simulink model "self_balancing_slink"  (R2023b)
settings: Solver=ode45  StartTime=0.0  StopTime=10.0  FixedStep=0.01  RelTol=0.001
values from neighbouring files (symbols this model uses):
  dt = 0.01    [bot_main.m]    (also in modelStateTransitionFcn.m)
  g = 9.81    [bot_main.m]    (also in eq_states.m; modelStateTransitionFcn.m)
  I_pend = 0.055    [bot_main.m]    (also in eq_states.m; modelStateTransitionFcn.m)
  Kd = Kg_d(i)    [bot_main.m]
  Ki = Kg_i(i)    [bot_main.m]
  Kp = Kg_p(i)    [bot_main.m]
  l = 0.159    [bot_main.m]    (also in eq_states.m; modelStateTransitionFcn.m)
  m_cart = 0.558    [bot_main.m]    (also in eq_states.m; modelStateTransitionFcn.m)
  m_pend = 1.267    [bot_main.m]    (also in eq_states.m; modelStateTransitionFcn.m)
  mu_drag = 0.00002    (= 2e-05)    [bot_main.m]    (also in eq_states.m = 0.2; modelStateTransitionFcn.m)
  noise_s1_value = np1(i)    [bot_main.m]
  noise_s2_value = np2(i)    [bot_main.m]
  x_init = [0; 0; (11/12)*pi; 0]    [bot_main.m]
libraries: simulink x4, slpidlib x2, sharedTrackingLibrary x2
settings Model: Creator=goate  LastModifiedBy=goate
settings SolverCC: ConsecutiveZCsStepRelTol=2.8421709430404e-13

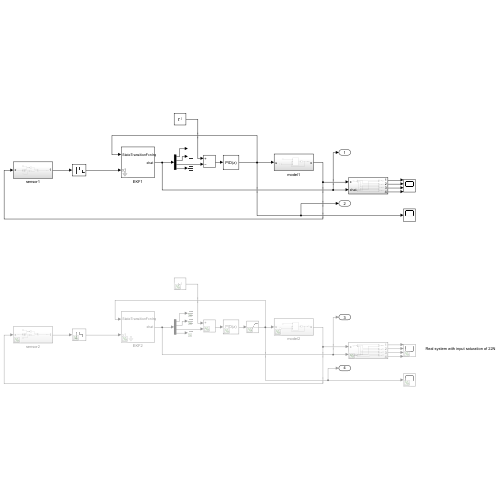
[thumbnail: Simulink's stored preview of the top-level diagram]
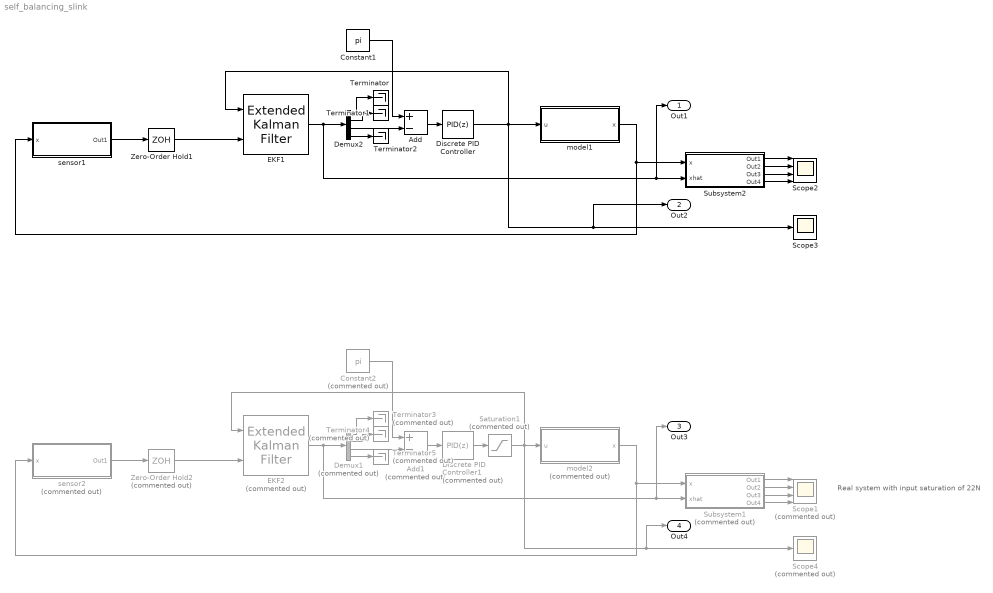
== system self_balancing_slink ==
  note: Real system with input saturation of 22N
  Add : Sum  Inputs=+-
  Add1 : Sum  Commented=on  Inputs=+-
  Constant1 : Constant  Value=pi
  Constant2 : Constant  Commented=on  Value=pi
  Demux1 : Demux  Commented=on
  Demux2 : Demux
  Discrete PID Controller : slpidlib/PID Controller  Controller=PID  Form=Parallel  TimeDomain=Discrete-time  UseExternalTs=off  SampleTime=dt  IntegratorMethod=Forward Euler  FilterMethod=Forward Euler  ControllerParametersSource=internal  P=Kp  I=Ki  UseKiTs=off  D=Kd  N=100  UseFilter=on  TunerSelectOption=Frequency Response Based  InitialConditionSource=internal  InitialConditionForIntegrator=0  InitialConditionForFilter=0  DifferentiatorICPrevScaledInput=0  ExternalReset=none  TrackingMode=off  Kt=1  LimitOutput=off  SatLimitsSource=internal  UpperSaturationLimit=inf  LowerSaturationLimit=-inf  LinearizeAsGain=off  AntiWindupMode=none  Kb=1  LimitIntegrator=off  UpperIntegratorSaturationLimit=inf  LowerIntegratorSaturationLimit=-inf  POutMin=[]  POutMax=[]  IOutMin=[]  IOutMax=[]  DOutMin=[]  DOutMax=[]  NOutMin=[]  NOutMax=[]  SumOutMin=[]  SumOutMax=[]  SaturationOutMin=[]  SaturationOutMax=[]  PParamMin=[]  PParamMax=[]  IParamMin=[]  IParamMax=[]  DParamMin=[]  DParamMax=[]  NParamMin=[]  NParamMax=[]  KbParamMin=[]  KbParamMax=[]  KtParamMin=[]  KtParamMax=[]  KbOutMin=[]  KbOutMax=[]  KtOutMin=[]  KtOutMax=[]  IntegratorOutMin=[]  IntegratorOutMax=[]  FilterOutMin=[]  FilterOutMax=[]  SumI1OutMin=[]  SumI1OutMax=[]  SumI2OutMin=[]  SumI2OutMax=[]  SumI3OutMin=[]  SumI3OutMax=[]  SumI4OutMin=[]  SumI4OutMax=[]  SumDOutMin=[]  SumDOutMax=[]  DifferentiatorOutMin=[]  DifferentiatorOutMax=[]  FilterDiffOutCoefMin=[]  FilterDiffOutCoefMax=[]  ReciprocalOutMin=[]  ReciprocalOutMax=[]  SumDenOutMin=[]  SumDenOutMax=[]  SumNumOutMin=[]  SumNumOutMax=[]  DivideOutMin=[]  DivideOutMax=[]  UdiffTsProdOutMin=[]  UdiffTsProdOutMax=[]  NTsProdOutMin=[]  NTsProdOutMax=[]  UintegralTsProdOutMin=[]  UintegralTsProdOutMax=[]  UngainTsProdOutMin=[]  UngainTsProdOutMax=[]  ClampingZeroOutDataTypeStr=Inherit: Inherit via back propagation  ClampingZeroOutMin=[]  ClampingZeroOutMax=[]  FilterDenConstantOutDataTypeStr=Inherit: Inherit via back propagation  FilterDenConstantOutMin=[]  FilterDenConstantOutMax=[]  PCopyOutDataTypeStr=Inherit: Inherit via back propagation  PCopyOutMin=[]  PCopyOutMax=[]  NCopyOutDataTypeStr=Inherit: Inherit via back propagation  NCopyOutMin=[]  NCopyOutMax=[]  IntegratorContinuousStateAttributes=''  IntegratorStateMustResolveToSignalObject=off  IntegratorRTWStateStorageClass=Auto  FilterContinuousStateAttributes=''  FilterStateMustResolveToSignalObject=off  FilterRTWStateStorageClass=Auto  ParallelPVariant=InternalParameters  IdealPVariant=Disabled  IVariant=InternalParameters  DVariant=InternalParameters  IntegratorVariant=Discrete  SatVariant=Disabled  AWVariant=Passthrough  PCopyVariant=Disabled  TRVariant=Disabled  FdbkBlocksVariant=Forward  IdealPFdbkVariant=Disabled  SatFdbkVariant=Disabled  DerivativeFilterVariant=ForwardEulerFilter  NVariant=InternalParameters  NCopyVariant=Disabled  FilterICVariant=InternalICsFilter  IntegratorICVariant=InternalICs  ExternalResetVariant=Disabled  TRSumVariant=Passthrough  SumFdbkVariant=Disabled  SumVariant=Sum_PID  TsampFilterVariant=InternalTs  TsampNgainVariant=Passthrough  TsampIntegralVariant=Disabled_SignalSpec  ExternalSaturationOutDataTypeStr=Inherit: Same as second input
      settings: LibrarySourceBlock=simulink/Discrete/Discrete PID Controller
  Discrete PID Controller1 : slpidlib/PID Controller  Commented=on  Controller=PID  Form=Parallel  TimeDomain=Discrete-time  UseExternalTs=off  SampleTime=dt  IntegratorMethod=Forward Euler  FilterMethod=Forward Euler  ControllerParametersSource=internal  P=Kp  I=Ki  UseKiTs=off  D=Kd  N=100  UseFilter=on  TunerSelectOption=Frequency Response Based  InitialConditionSource=internal  InitialConditionForIntegrator=0  InitialConditionForFilter=0  DifferentiatorICPrevScaledInput=0  ExternalReset=none  TrackingMode=off  Kt=1  LimitOutput=off  SatLimitsSource=internal  UpperSaturationLimit=inf  LowerSaturationLimit=-inf  LinearizeAsGain=off  AntiWindupMode=none  Kb=1  LimitIntegrator=off  UpperIntegratorSaturationLimit=inf  LowerIntegratorSaturationLimit=-inf  POutMin=[]  POutMax=[]  IOutMin=[]  IOutMax=[]  DOutMin=[]  DOutMax=[]  NOutMin=[]  NOutMax=[]  SumOutMin=[]  SumOutMax=[]  SaturationOutMin=[]  SaturationOutMax=[]  PParamMin=[]  PParamMax=[]  IParamMin=[]  IParamMax=[]  DParamMin=[]  DParamMax=[]  NParamMin=[]  NParamMax=[]  KbParamMin=[]  KbParamMax=[]  KtParamMin=[]  KtParamMax=[]  KbOutMin=[]  KbOutMax=[]  KtOutMin=[]  KtOutMax=[]  IntegratorOutMin=[]  IntegratorOutMax=[]  FilterOutMin=[]  FilterOutMax=[]  SumI1OutMin=[]  SumI1OutMax=[]  SumI2OutMin=[]  SumI2OutMax=[]  SumI3OutMin=[]  SumI3OutMax=[]  SumI4OutMin=[]  SumI4OutMax=[]  SumDOutMin=[]  SumDOutMax=[]  DifferentiatorOutMin=[]  DifferentiatorOutMax=[]  FilterDiffOutCoefMin=[]  FilterDiffOutCoefMax=[]  ReciprocalOutMin=[]  ReciprocalOutMax=[]  SumDenOutMin=[]  SumDenOutMax=[]  SumNumOutMin=[]  SumNumOutMax=[]  DivideOutMin=[]  DivideOutMax=[]  UdiffTsProdOutMin=[]  UdiffTsProdOutMax=[]  NTsProdOutMin=[]  NTsProdOutMax=[]  UintegralTsProdOutMin=[]  UintegralTsProdOutMax=[]  UngainTsProdOutMin=[]  UngainTsProdOutMax=[]  ClampingZeroOutDataTypeStr=Inherit: Inherit via back propagation  ClampingZeroOutMin=[]  ClampingZeroOutMax=[]  FilterDenConstantOutDataTypeStr=Inherit: Inherit via back propagation  FilterDenConstantOutMin=[]  FilterDenConstantOutMax=[]  PCopyOutDataTypeStr=Inherit: Inherit via back propagation  PCopyOutMin=[]  PCopyOutMax=[]  NCopyOutDataTypeStr=Inherit: Inherit via back propagation  NCopyOutMin=[]  NCopyOutMax=[]  IntegratorContinuousStateAttributes=''  IntegratorStateMustResolveToSignalObject=off  IntegratorRTWStateStorageClass=Auto  FilterContinuousStateAttributes=''  FilterStateMustResolveToSignalObject=off  FilterRTWStateStorageClass=Auto  ParallelPVariant=InternalParameters  IdealPVariant=Disabled  IVariant=InternalParameters  DVariant=InternalParameters  IntegratorVariant=Discrete  SatVariant=Disabled  AWVariant=Passthrough  PCopyVariant=Disabled  TRVariant=Disabled  FdbkBlocksVariant=Forward  IdealPFdbkVariant=Disabled  SatFdbkVariant=Disabled  DerivativeFilterVariant=ForwardEulerFilter  NVariant=InternalParameters  NCopyVariant=Disabled  FilterICVariant=InternalICsFilter  IntegratorICVariant=InternalICs  ExternalResetVariant=Disabled  TRSumVariant=Passthrough  SumFdbkVariant=Disabled  SumVariant=Sum_PID  TsampFilterVariant=InternalTs  TsampNgainVariant=Passthrough  TsampIntegralVariant=Disabled_SignalSpec  ExternalSaturationOutDataTypeStr=Inherit: Same as second input
      settings: LibrarySourceBlock=simulink/Discrete/Discrete PID Controller
  EKF1 : sharedTrackingLibrary/Extended Kalman Filter  StateTransitionFcn=modelStateTransitionFcn  HasStateTransitionJacobianFcn=off  HasAdditiveProcessNoise=Additive  ProcessNoise=0  HasTimeVaryingProcessNoise=off  HasStateTransitionFcnExtraArgument=1  InitialState=x_init  InitialStateCovariance=initial_cov  MeasurementFcn1=modelMeasureFcn  HasMeasurementJacobianFcn1=off  HasMeasurementEnablePort1=off  HasAdditiveMeasurementNoise1=Additive  MeasurementNoise1=measurement_cov  HasTimeVaryingMeasurementNoise1=off  HasMeasurementFcnExtraArgument1=0  HasMeasurementWrapping1=off  MeasurementFcn2=myMeasurementFcn  HasMeasurementJacobianFcn2=off  HasMeasurementEnablePort2=off  HasAdditiveMeasurementNoise2=Additive  MeasurementNoise2=1  HasTimeVaryingMeasurementNoise2=off  HasMeasurementFcnExtraArgument2=0  HasMeasurementWrapping2=off  MeasurementFcn3=myMeasurementFcn  HasMeasurementJacobianFcn3=off  HasMeasurementEnablePort3=off  HasAdditiveMeasurementNoise3=Additive  MeasurementNoise3=1  HasTimeVaryingMeasurementNoise3=off  HasMeasurementFcnExtraArgument3=0  HasMeasurementWrapping3=off  MeasurementFcn4=myMeasurementFcn  HasMeasurementJacobianFcn4=off  HasMeasurementEnablePort4=off  HasAdditiveMeasurementNoise4=Additive  MeasurementNoise4=1  HasTimeVaryingMeasurementNoise4=off  HasMeasurementFcnExtraArgument4=0  HasMeasurementWrapping4=off  MeasurementFcn5=myMeasurementFcn  HasMeasurementJacobianFcn5=off  HasMeasurementEnablePort5=off  HasAdditiveMeasurementNoise5=Additive  MeasurementNoise5=1  HasTimeVaryingMeasurementNoise5=off  HasMeasurementFcnExtraArgument5=0  HasMeasurementWrapping5=off  EnableMultirate=off  StateTransitionFcnSampleTime=1  MeasurementFcn1SampleTime=1  MeasurementFcn2SampleTime=1  MeasurementFcn3SampleTime=1  MeasurementFcn4SampleTime=1  MeasurementFcn5SampleTime=1  UseCurrentEstimator=on  OutputStateCovariance=off  DataType=double  SampleTime=dt  NumberOfMeasurements=1
  EKF2 : sharedTrackingLibrary/Extended Kalman Filter  Commented=on  StateTransitionFcn=modelStateTransitionFcn  HasStateTransitionJacobianFcn=off  HasAdditiveProcessNoise=Additive  ProcessNoise=0  HasTimeVaryingProcessNoise=off  HasStateTransitionFcnExtraArgument=1  InitialState=x_init  InitialStateCovariance=initial_cov  MeasurementFcn1=modelMeasureFcn  HasMeasurementJacobianFcn1=off  HasMeasurementEnablePort1=off  HasAdditiveMeasurementNoise1=Additive  MeasurementNoise1=measurement_cov  HasTimeVaryingMeasurementNoise1=off  HasMeasurementFcnExtraArgument1=0  HasMeasurementWrapping1=off  MeasurementFcn2=myMeasurementFcn  HasMeasurementJacobianFcn2=off  HasMeasurementEnablePort2=off  HasAdditiveMeasurementNoise2=Additive  MeasurementNoise2=1  HasTimeVaryingMeasurementNoise2=off  HasMeasurementFcnExtraArgument2=0  HasMeasurementWrapping2=off  MeasurementFcn3=myMeasurementFcn  HasMeasurementJacobianFcn3=off  HasMeasurementEnablePort3=off  HasAdditiveMeasurementNoise3=Additive  MeasurementNoise3=1  HasTimeVaryingMeasurementNoise3=off  HasMeasurementFcnExtraArgument3=0  HasMeasurementWrapping3=off  MeasurementFcn4=myMeasurementFcn  HasMeasurementJacobianFcn4=off  HasMeasurementEnablePort4=off  HasAdditiveMeasurementNoise4=Additive  MeasurementNoise4=1  HasTimeVaryingMeasurementNoise4=off  HasMeasurementFcnExtraArgument4=0  HasMeasurementWrapping4=off  MeasurementFcn5=myMeasurementFcn  HasMeasurementJacobianFcn5=off  HasMeasurementEnablePort5=off  HasAdditiveMeasurementNoise5=Additive  MeasurementNoise5=1  HasTimeVaryingMeasurementNoise5=off  HasMeasurementFcnExtraArgument5=0  HasMeasurementWrapping5=off  EnableMultirate=off  StateTransitionFcnSampleTime=1  MeasurementFcn1SampleTime=1  MeasurementFcn2SampleTime=1  MeasurementFcn3SampleTime=1  MeasurementFcn4SampleTime=1  MeasurementFcn5SampleTime=1  UseCurrentEstimator=on  OutputStateCovariance=off  DataType=double  SampleTime=dt  NumberOfMeasurements=1
  Saturation1 : Saturate  Commented=on  UpperLimit=22  LowerLimit=-22
  Scope1 : Scope  Commented=on  NumInputPorts=4
  Scope2 : Scope  NumInputPorts=4
  Scope3 : Scope
  Scope4 : Scope  Commented=on
  Subsystem1 : Subsystem  Commented=on
  Subsystem2 : Subsystem
  Terminator : Terminator
  Terminator1 : Terminator
  Terminator2 : Terminator
  Terminator3 : Terminator  Commented=on
  Terminator4 : Terminator  Commented=on
  Terminator5 : Terminator  Commented=on
  Zero-Order Hold1 : ZeroOrderHold  SampleTime=dt
  Zero-Order Hold2 : ZeroOrderHold  Commented=on  SampleTime=dt
  model1 : Subsystem
  model2 : Subsystem  Commented=on
  sensor1 : Subsystem
  sensor2 : Subsystem  Commented=on
  Out1 : Outport
  Out2 : Outport  Port=2
  Out3 : Outport  Port=3
  Out4 : Outport  Port=4
  wires:
  sensor1/1(Out1) -> Zero-Order Hold1/1
  Zero-Order Hold1/1 -> EKF1/2
  model1/1(x) -> Subsystem2/1(x), sensor1/1(x)
  EKF1/1 -> Out1/1, Subsystem2/2(xhat), Demux2/1
  Demux2/1 -> Terminator/1
  Demux2/4 -> Terminator2/1
  Demux2/2 -> Terminator1/1
  Demux2/3 -> Add/2
  Constant1/1 -> Add/1
  Add/1 -> Discrete PID Controller/1
  Subsystem2/1(Out1) -> Scope2/1
  Subsystem2/2(Out2) -> Scope2/2
  Subsystem2/3(Out3) -> Scope2/3
  Subsystem2/4(Out4) -> Scope2/4
  Discrete PID Controller1/1 -> Saturation1/1
  model2/1(x) -> Subsystem1/1(x), sensor2/1(x)
  Zero-Order Hold2/1 -> EKF2/2
  Subsystem1/4(Out4) -> Scope1/4
  Subsystem1/3(Out3) -> Scope1/3
  Subsystem1/2(Out2) -> Scope1/2
  Subsystem1/1(Out1) -> Scope1/1
  Add1/1 -> Discrete PID Controller1/1
  Constant2/1 -> Add1/1
  sensor2/1(Out1) -> Zero-Order Hold2/1
  Demux1/1 -> Terminator3/1
  Demux1/3 -> Add1/2
  EKF2/1 -> Out3/1, Subsystem1/2(xhat), Demux1/1
  Saturation1/1 -> EKF2/1, Out4/1, Scope4/1, model2/1(u)
  Demux1/2 -> Terminator4/1
  Demux1/4 -> Terminator5/1
  Discrete PID Controller/1 -> EKF1/1, Out2/1, Scope3/1, model1/1(u)

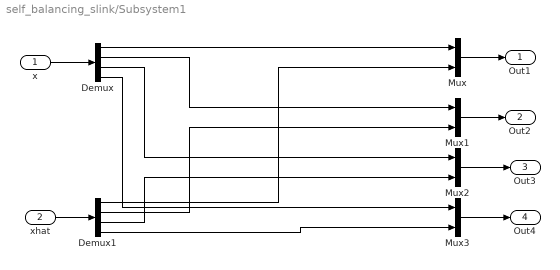
== system self_balancing_slink/Subsystem1 ==
  x : Inport
  xhat : Inport  Port=2
  Demux : Demux
  Demux1 : Demux
  Mux{,1..3} (4 alike) : Mux  Inputs=2
  Out1 : Outport
  Out2 : Outport  Port=2
  Out3 : Outport  Port=3
  Out4 : Outport  Port=4
  wires:
  x/1 -> Demux/1
  xhat/1 -> Demux1/1
  Demux/1 -> Mux/1
  Mux/1 -> Out1/1
  Demux1/1 -> Mux/2
  Mux1/1 -> Out2/1
  Demux1/2 -> Mux1/2
  Demux/2 -> Mux1/1
  Demux1/3 -> Mux2/2
  Demux/3 -> Mux2/1
  Mux2/1 -> Out3/1
  Mux3/1 -> Out4/1
  Demux1/4 -> Mux3/2
  Demux/4 -> Mux3/1

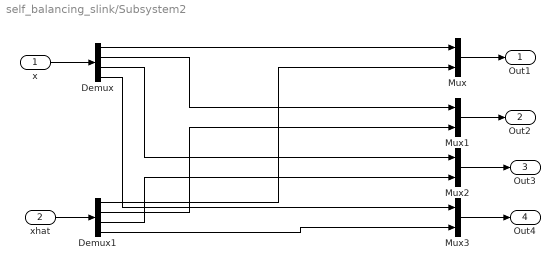
== system self_balancing_slink/Subsystem2 ==
  x : Inport
  xhat : Inport  Port=2
  Demux : Demux
  Demux1 : Demux
  Mux{,1..3} (4 alike) : Mux  Inputs=2
  Out1 : Outport
  Out2 : Outport  Port=2
  Out3 : Outport  Port=3
  Out4 : Outport  Port=4
  wires:
  x/1 -> Demux/1
  xhat/1 -> Demux1/1
  Demux/1 -> Mux/1
  Mux/1 -> Out1/1
  Demux1/1 -> Mux/2
  Mux1/1 -> Out2/1
  Demux1/2 -> Mux1/2
  Demux/2 -> Mux1/1
  Demux1/3 -> Mux2/2
  Demux/3 -> Mux2/1
  Mux2/1 -> Out3/1
  Mux3/1 -> Out4/1
  Demux1/4 -> Mux3/2
  Demux/4 -> Mux3/1

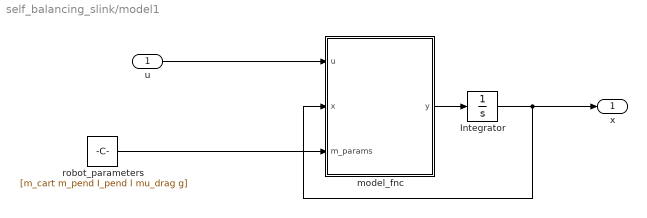
== system self_balancing_slink/model1 ==
  u : Inport
  Integrator : Integrator  InitialCondition=x_init
  model_fnc : MATLAB Function  TreatAsAtomicUnit=on
  robot_parameters : Constant  Value=[m_cart m_pend I_pend l mu_drag g]
  x : Outport
  wires:
  u/1 -> model_fnc/1(u)
  robot_parameters/1 -> model_fnc/3(m_params)
  model_fnc/1(y) -> Integrator/1
  Integrator/1 -> model_fnc/2(x), x/1

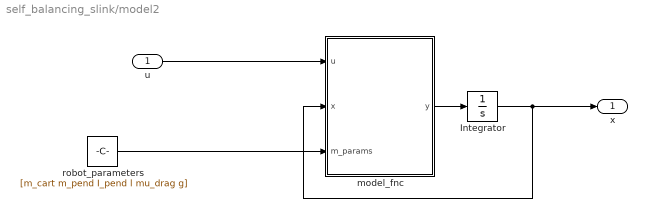
== system self_balancing_slink/model2 ==
  u : Inport
  Integrator : Integrator  InitialCondition=x_init
  model_fnc : MATLAB Function  TreatAsAtomicUnit=on
  robot_parameters : Constant  Value=[m_cart m_pend I_pend l mu_drag g]
  x : Outport
  wires:
  u/1 -> model_fnc/1(u)
  robot_parameters/1 -> model_fnc/3(m_params)
  model_fnc/1(y) -> Integrator/1
  Integrator/1 -> model_fnc/2(x), x/1

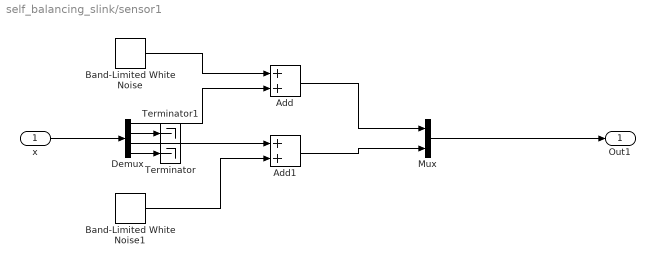
== system self_balancing_slink/sensor1 ==
  x : Inport
  Add : Sum
  Add1 : Sum
  Band-Limited White Noise : simulink/Sources/Band-Limited White Noise  Cov=[noise_s1_value]  Ts=dt  seed=[23341]
  Band-Limited White Noise1 : simulink/Sources/Band-Limited White Noise  Cov=[noise_s2_value]  Ts=dt  seed=[23341]
  Demux : Demux
  Mux : Mux  Inputs=2
  Terminator : Terminator
  Terminator1 : Terminator
  Out1 : Outport
  wires:
  x/1 -> Demux/1
  Band-Limited White Noise/1 -> Add/1
  Demux/1 -> Add/2
  Demux/3 -> Add1/1
  Band-Limited White Noise1/1 -> Add1/2
  Demux/4 -> Terminator/1
  Demux/2 -> Terminator1/1
  Add/1 -> Mux/1
  Add1/1 -> Mux/2
  Mux/1 -> Out1/1

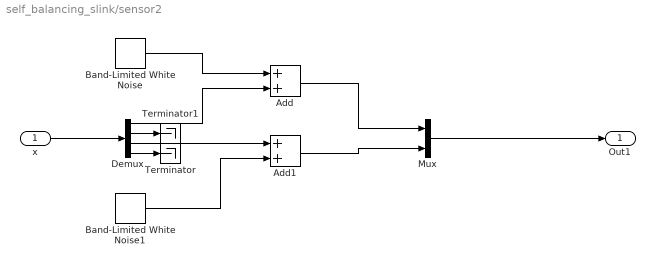
== system self_balancing_slink/sensor2 ==
  x : Inport
  Add : Sum
  Add1 : Sum
  Band-Limited White Noise : simulink/Sources/Band-Limited White Noise  Cov=[noise_s1_value]  Ts=dt  seed=[23341]
  Band-Limited White Noise1 : simulink/Sources/Band-Limited White Noise  Cov=[noise_s2_value]  Ts=dt  seed=[23341]
  Demux : Demux
  Mux : Mux  Inputs=2
  Terminator : Terminator
  Terminator1 : Terminator
  Out1 : Outport
  wires:
  x/1 -> Demux/1
  Band-Limited White Noise/1 -> Add/1
  Demux/1 -> Add/2
  Demux/3 -> Add1/1
  Band-Limited White Noise1/1 -> Add1/2
  Demux/4 -> Terminator/1
  Demux/2 -> Terminator1/1
  Add/1 -> Mux/1
  Add1/1 -> Mux/2
  Mux/1 -> Out1/1

== matlab function self_balancing_slink/model2/model_fnc ==
  data: u input; y output; x input; m_params input
function y = fcn(u, x, m_params)

% This is the model without any measurement noise, we'll add it afterwards

% IN THIS MODEL THE EQUATION UNSTABLE EQUILIBRIUM POINT IS [0, 0, PI, 0]
% WHILE THE STABLE ONE IS [0, 0, 0, 0].

m_cart = m_params(1);
m_pend = m_params(2);
I_pend = m_params(3);
l = m_params(4);
mu_drag = m_params(5);
g = m_params(6);

m_tot = m_cart + m_pend;

dx1 = x(2);
dx2 = (u - mu_drag*x(2) - m_pend*l*(((-m_pend*g*l*sin(x(3))*cos(x(3)))/(I_pend + m_pend*l^2)) - (x(4)^2)*sin(x(3))))/...
    (m_tot*(1 - (((m_pend^2)*(l^2)*(cos(x(3))^2))/(I_pend + m_pend*l^2))));
dx3 = x(4);
dx4 = (-m_pend*g*l*sin(x(3)) -m_pend*l*dx2*cos(x(3)))/(I_pend + m_pend*l^2);

xddot = [
  dx1;
  dx2;
  dx3;
  dx4
];

y = xddot;

== matlab function self_balancing_slink/model1/model_fnc ==
  data: u input; y output; x input; m_params input
function y = fcn(u, x, m_params)

% This is the model without any measurement noise, we'll add it afterwards

% IN THIS MODEL THE EQUATION UNSTABLE EQUILIBRIUM POINT IS [0, 0, PI, 0]
% WHILE THE STABLE ONE IS [0, 0, 0, 0].

m_cart = m_params(1);
m_pend = m_params(2);
I_pend = m_params(3);
l = m_params(4);
mu_drag = m_params(5);
g = m_params(6);

m_tot = m_cart + m_pend;

dx1 = x(2);
dx2 = (u - mu_drag*x(2) - m_pend*l*(((-m_pend*g*l*sin(x(3))*cos(x(3)))/(I_pend + m_pend*l^2)) - (x(4)^2)*sin(x(3))))/...
    (m_tot*(1 - (((m_pend^2)*(l^2)*(cos(x(3))^2))/(I_pend + m_pend*l^2))));
dx3 = x(4);
dx4 = (-m_pend*g*l*sin(x(3)) -m_pend*l*dx2*cos(x(3)))/(I_pend + m_pend*l^2);

xddot = [
  dx1;
  dx2;
  dx3;
  dx4
];

y = xddot;
